simulink model "slezh_sost_all"  (R2024a)
settings: Solver=FixedStepAuto  StartTime=0.0  StopTime=5  FixedStep=0.0001  RelTol=1e-3
values from neighbouring files (symbols this model uses):
  A = [11 -2 13; 6 -1 6; -6 -1 -8]    [comp_sost.m]    (also in meandr.m = [0 1; 0 0]; out.m; out_copy.m; rank_extended.m)
  B = [2; 0; 0]    [comp_sost.m]    (also in meandr.m = [0; 1]; out.m; out_copy.m; slezh_sost.m)
  Cz = [-2 3 -1]    [comp_sost.m]    (also in meandr.m = -C; out.m; out_copy.m = C; slezh_sost.m)
  Dz = 16/pi * [1 0 1/3 0 1/5 0]    [meandr.m]    (also in out.m = [3 4 2 -3]; out_copy.m = D; slezh_sost.m = [3 4 2 -3])
  G = [35 56 22 -42; -11 -17 -7 12; -6 -10 -5 10; 11 18 6 -13]    [comp_sost.m]    (also in meandr.m = [0 1 0 0 0 0; -1 0 0 0 0 0; 0 0 0 3 0 0; 0 0 -3 0 0 0; 0 0 0; out.m; out_copy.m; rank_extended.m)
  K1 = -inv(R)*B'*P    [comp_sost.m]    (also in meandr.m; out.m = -R\B'*P; out_copy.m; slezh_sost.m)
  K2 = double(Y_sol - K1*P_sol)    [comp_sost.m]    (also in meandr.m; out.m; out_copy.m; slezh_sost.m)
settings Model: Creator=ventus  LastModifiedBy=ventus

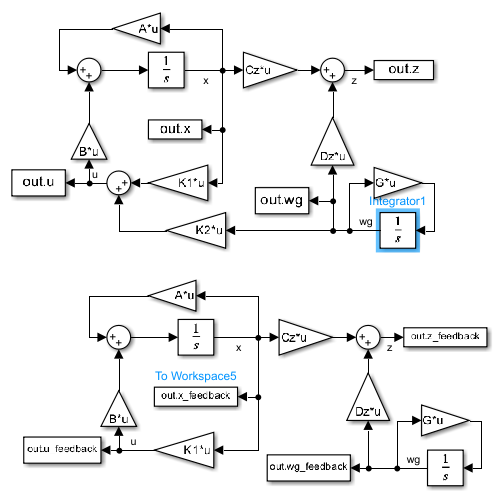
[thumbnail: Simulink's stored preview of the top-level diagram]
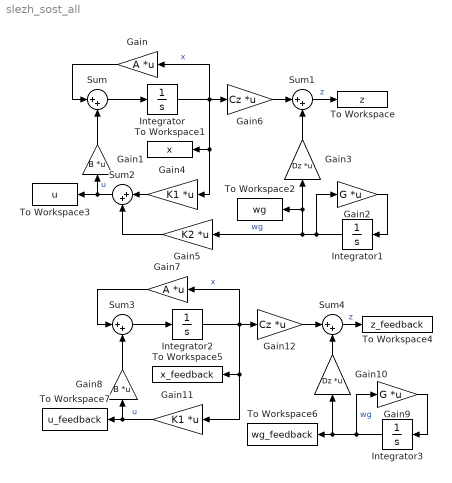
== system slezh_sost_all ==
  Gain : Gain  Gain=A  Multiplication=Matrix(K*u)
  Gain1 : Gain  Gain=B  Multiplication=Matrix(K*u)
  Gain10 : Gain  Gain=Dz  Multiplication=Matrix(K*u)
  Gain11 : Gain  Gain=K1  Multiplication=Matrix(K*u)
  Gain12 : Gain  Gain=Cz  Multiplication=Matrix(K*u)
  Gain2 : Gain  Gain=G  Multiplication=Matrix(K*u)
  Gain3 : Gain  Gain=Dz  Multiplication=Matrix(K*u)
  Gain4 : Gain  Gain=K1  Multiplication=Matrix(K*u)
  Gain5 : Gain  Gain=K2  Multiplication=Matrix(K*u)
  Gain6 : Gain  Gain=Cz  Multiplication=Matrix(K*u)
  Gain7 : Gain  Gain=A  Multiplication=Matrix(K*u)
  Gain8 : Gain  Gain=B  Multiplication=Matrix(K*u)
  Gain9 : Gain  Gain=G  Multiplication=Matrix(K*u)
  Integrator : Integrator  InitialCondition=[1; 1; 1]
  Integrator1 : Integrator  InitialCondition=[1; 1; 1; 1]
  Integrator2 : Integrator  InitialCondition=[1; 1; 1]
  Integrator3 : Integrator  InitialCondition=[1; 1; 1; 1]
  Sum{,1..4} (5 alike) : Sum  Inputs=|++
  To Workspace : ToWorkspace  VariableName=z  SaveFormat=Timeseries  SampleTime=-1
  To Workspace1 : ToWorkspace  VariableName=x  SaveFormat=Timeseries  SampleTime=-1
  To Workspace2 : ToWorkspace  VariableName=wg  SaveFormat=Timeseries  SampleTime=-1
  To Workspace3 : ToWorkspace  VariableName=u  SaveFormat=Timeseries  SampleTime=-1
  To Workspace4 : ToWorkspace  VariableName=z_feedback  SaveFormat=Timeseries  SampleTime=-1
  To Workspace5 : ToWorkspace  VariableName=x_feedback  SaveFormat=Timeseries  SampleTime=-1
  To Workspace6 : ToWorkspace  VariableName=wg_feedback  SaveFormat=Timeseries  SampleTime=-1
  To Workspace7 : ToWorkspace  VariableName=u_feedback  SaveFormat=Timeseries  SampleTime=-1
  wires:
  Gain1/1 -> Sum/2
  Gain4/1 -> Sum2/1
  Sum/1 -> Integrator/1
  Integrator/1 -> Gain6/1, Gain/1, Gain4/1, To Workspace1/1  "x"
  Gain3/1 -> Sum1/2
  Sum2/1 -> Gain1/1, To Workspace3/1  "u"
  Gain2/1 -> Integrator1/1
  Gain6/1 -> Sum1/1
  Sum1/1 -> To Workspace/1  "z"
  Integrator1/1 -> Gain2/1, To Workspace2/1, Gain3/1, Gain5/1  "wg"
  Gain/1 -> Sum/1
  Gain5/1 -> Sum2/2
  Integrator2/1 -> Gain12/1, Gain7/1, Gain11/1, To Workspace5/1  "x"
  Gain9/1 -> Integrator3/1
  Gain11/1 -> Gain8/1, To Workspace7/1  "u"
  Gain12/1 -> Sum4/1
  Gain8/1 -> Sum3/2
  Sum4/1 -> To Workspace4/1  "z"
  Sum3/1 -> Integrator2/1
  Gain10/1 -> Sum4/2
  Integrator3/1 -> Gain9/1, To Workspace6/1, Gain10/1  "wg"
  Gain7/1 -> Sum3/1
